simulink model "LookupTable"  (R2015b)
settings: Solver=VariableStepAuto  StartTime=0.0  StopTime=10.0  RelTol=1e-3
settings Model: Creator=LUBO  LastModifiedBy=LUBO

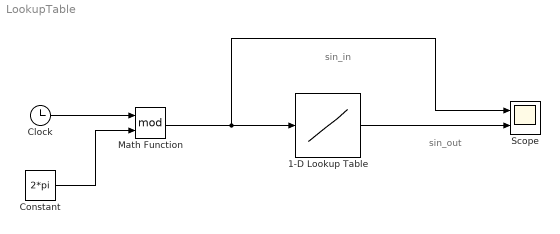
== system LookupTable ==
  note: sin_out
  note: sin_in
  1-D Lookup Table : Lookup_n-D  NumberOfTableDimensions=1  BreakpointsForDimension1=linspace(0,2*pi,256)  Table=sin(linspace(0,2*pi,256))  InternalRulePriority=Speed  RndMeth=Simplest  InputSameDT=on
  Clock : Clock
  Constant : Constant  Value=2*pi
  Math Function : Math  Operator=mod  SaturateOnIntegerOverflow=on
  Scope : Scope  NumInputPorts=2
  wires:
  Clock/1 -> Math Function/1
  Constant/1 -> Math Function/2
  Math Function/1 -> Scope/1, 1-D Lookup Table/1
  1-D Lookup Table/1 -> Scope/2
